simulink model "dof14model_rev"  (R2024a)
settings: Solver=ode4  StartTime=0.0  StopTime=simtime  FixedStep=samtime  RelTol=1e-3
values from neighbouring files (symbols this model uses):
  a = data(n,2)    [main_dof14model.m]
  b = data(n,3)    [main_dof14model.m]
  Csfl = data(n,22)    [main_dof14model.m]
  Csfr = data(n,23)    [main_dof14model.m]
  Csrl = data(n,24)    [main_dof14model.m]
  Csrr = data(n,25)    [main_dof14model.m]
  h = data(n,6)    [main_dof14model.m]
  Ip = data(n,10)    [main_dof14model.m]
  Ir = data(n,11)    [main_dof14model.m]
  Iw = data(n,17)    [main_dof14model.m]
  Jz = data(n,12)    [main_dof14model.m]
  Ksfl = data(n,18)    [main_dof14model.m]
  Ksfr = data(n,19)    [main_dof14model.m]
  Ksrl = data(n,20)    [main_dof14model.m]
  Ksrr = data(n,21)    [main_dof14model.m]
  Ktfl = data(n,28)    [main_dof14model.m]
  Ktfr = data(n,29)    [main_dof14model.m]
  Ktrl = data(n,30)    [main_dof14model.m]
  Ktrr = data(n,31)    [main_dof14model.m]
  Lf = data(n,8)    [main_dof14model.m]
  Lr = data(n,9)    [main_dof14model.m]
  Ms = data(n,1)    [main_dof14model.m]
  mt = data(n,7)    [main_dof14model.m]
  mufl = data(n,13)    [main_dof14model.m]
  mufr = data(n,14)    [main_dof14model.m]
  murl = data(n,15)    [main_dof14model.m]
  murr = data(n,16)    [main_dof14model.m]
  Rw = data(n,27)    [main_dof14model.m]
  wf = data(n,4)    [main_dof14model.m]
  wr = data(n,5)    [main_dof14model.m]
undefined symbols (not defined in the file or in its folder): sigbuilder_block
(part 2 of 2)

== system dof14model_rev/Subsys Tire/Subsys tfl1/Subsys Fy ==
  note: Sh
  note: x
  note: X
  note: Bx - atanBX
  note: Bx
  note: B
  alpha : Inport
  Fz : Inport  Port=2
  Bx : Product  RndMeth=Zero
  C : Constant  Value=1.3
  Divide : Product  Inputs=*/
  Product{1..4} (4 alike) : Product  RndMeth=Zero
  Scope2 : Scope
  Subsys BCD : Subsystem
  Subsys D : Subsystem
  SubsysE : Subsystem
  Subtract : Sum  Inputs=+-
  Subtract1 : Sum  Inputs=+-
  Subtract3 : Sum
  Subtract4 : Sum
  Sv : Constant  Value=0
  Sv1 : Constant  Value=0
  To Workspace1 : ToWorkspace  VariableName=Fyfrs  SampleTime=-1
  atan : Trigonometry  Operator=atan
  atanBx : Trigonometry  Operator=atan
  atanBx1 : Trigonometry
  Fy : Outport
  wires:
  Fz/1 -> SubsysE/1(Fz), Subsys D/1(Fz), Subsys BCD/1(Fz)
  alpha/1 -> Subtract4/1
  Subsys BCD/1(BCD) -> Divide/1
  Sv1/1 -> Subtract4/2
  Divide/1 -> Bx/2
  Bx/1 -> atanBx/1, Subtract1/1, Subtract/1
  atanBx/1 -> Subtract/2
  Subtract/1 -> Product1/1
  SubsysE/1(E) -> Product1/2
  Product1/1 -> Subtract1/2
  Subtract1/1 -> atan/1
  Sv/1 -> Subtract3/2
  Subtract4/1 -> Bx/1
  atan/1 -> Product3/1
  atanBx1/1 -> Product4/1
  Product3/1 -> atanBx1/1
  Product4/1 -> Subtract3/1
  Subtract3/1 -> Fy/1, To Workspace1/1, Scope2/1
  Product2/1 -> Divide/2
  Subsys D/1(D) -> Product4/2, Product2/2
  C/1 -> Product3/2, Product2/1

== system dof14model_rev/Subsys Tire/Subsys tfl1/Subsys Mz ==
  note: x
  note: X
  note: Bx - atanBX
  note: Bx
  note: B
  alpha : Inport
  Fz : Inport  Port=2
  Bx : Product  RndMeth=Zero
  C : Constant  Value=2.40
  Divide : Product  Inputs=*/
  Product{1..4} (4 alike) : Product  RndMeth=Zero
  Scope2 : Scope
  Sh2 : Constant  Value=0
  Subsys BCD : Subsystem
  Subsys D : Subsystem
  SubsysE : Subsystem
  Subtract : Sum  Inputs=+-
  Subtract1 : Sum  Inputs=+-
  Subtract3 : Sum
  Subtract4 : Sum
  Sv2 : Constant  Value=0
  To Workspace1 : ToWorkspace  VariableName=Mzfrs  SampleTime=-1
  atan : Trigonometry  Operator=atan
  atanBx : Trigonometry  Operator=atan
  atanBx1 : Trigonometry
  Mz : Outport
  wires:
  Fz/1 -> SubsysE/1(Fz), Subsys D/1(Fz), Subsys BCD/1(Fz)
  Sh2/1 -> Subtract4/2
  Divide/1 -> Bx/2
  Bx/1 -> atanBx/1, Subtract1/1, Subtract/1
  atanBx/1 -> Subtract/2
  Subtract/1 -> Product1/1
  SubsysE/1(E) -> Product1/2
  Product1/1 -> Subtract1/2
  Subtract1/1 -> atan/1
  Sv2/1 -> Subtract3/2
  Subtract4/1 -> Bx/1
  alpha/1 -> Subtract4/1
  atan/1 -> Product3/1
  atanBx1/1 -> Product4/1
  Product3/1 -> atanBx1/1
  Product4/1 -> Subtract3/1
  Subtract3/1 -> Mz/1, To Workspace1/1, Scope2/1
  Product2/1 -> Divide/2
  Subsys BCD/1(BCD) -> Divide/1
  Subsys D/1(D) -> Product4/2, Product2/2
  C/1 -> Product3/2, Product2/1

== system dof14model_rev/Subsys Tire/Subsys tfl2/Subsys Fx ==
  note: B
  note: Bx
  note: Bx - atanBX
  note: X
  note: x
  S : Inport
  Fz : Inport  Port=2
  Bx : Product  RndMeth=Zero
  C : Constant  Value=1.65
  Divide : Product  Inputs=*/
  Gain : Gain  Gain=100
  Product{1..4} (4 alike) : Product  RndMeth=Zero
  Scope2 : Scope
  Sh2 : Constant  Value=0
  Subsys BCD : Subsystem
  Subsys D : Subsystem
  SubsysE : Subsystem
  Subtract : Sum  Inputs=+-
  Subtract1 : Sum  Inputs=+-
  Subtract3 : Sum
  Subtract4 : Sum
  Sv : Constant  Value=0
  To Workspace1 : ToWorkspace  VariableName=Fxrls  SampleTime=-1
  atan : Trigonometry  Operator=atan
  atanBx : Trigonometry  Operator=atan
  atanBx1 : Trigonometry
  Fx : Outport
  wires:
  C/1 -> Product2/1, Product3/2
  Subsys D/1(D) -> Product2/2, Product4/2
  Subsys BCD/1(BCD) -> Divide/1
  Product2/1 -> Divide/2
  Subtract3/1 -> Scope2/1, To Workspace1/1, Fx/1
  Product4/1 -> Subtract3/1
  Product3/1 -> atanBx1/1
  atanBx1/1 -> Product4/1
  atan/1 -> Product3/1
  S/1 -> Gain/1
  Subtract4/1 -> Bx/1
  Sv/1 -> Subtract3/2
  Subtract1/1 -> atan/1
  Product1/1 -> Subtract1/2
  SubsysE/1(E) -> Product1/2
  Subtract/1 -> Product1/1
  atanBx/1 -> Subtract/2
  Bx/1 -> Subtract/1, Subtract1/1, atanBx/1
  Divide/1 -> Bx/2
  Sh2/1 -> Subtract4/2
  Fz/1 -> Subsys BCD/1(Fz), Subsys D/1(Fz), SubsysE/1(Fz)
  Gain/1 -> Subtract4/1

== system dof14model_rev/Subsys Tire/Subsys tfl2/Subsys Fy ==
  note: B
  note: Bx
  note: Bx - atanBX
  note: X
  note: x
  note: Sh
  alpha : Inport
  Fz : Inport  Port=2
  Bx : Product  RndMeth=Zero
  C : Constant  Value=1.3
  Divide : Product  Inputs=*/
  Product{1..4} (4 alike) : Product  RndMeth=Zero
  Scope2 : Scope
  Subsys BCD : Subsystem
  Subsys D : Subsystem
  SubsysE : Subsystem
  Subtract : Sum  Inputs=+-
  Subtract1 : Sum  Inputs=+-
  Subtract3 : Sum
  Subtract4 : Sum
  Sv : Constant  Value=0
  Sv1 : Constant  Value=0
  To Workspace1 : ToWorkspace  VariableName=Fyrls  SampleTime=-1
  atan : Trigonometry  Operator=atan
  atanBx : Trigonometry  Operator=atan
  atanBx1 : Trigonometry
  Fy : Outport
  wires:
  C/1 -> Product2/1, Product3/2
  Subsys D/1(D) -> Product2/2, Product4/2
  Product2/1 -> Divide/2
  Subtract3/1 -> Scope2/1, To Workspace1/1, Fy/1
  Product4/1 -> Subtract3/1
  Product3/1 -> atanBx1/1
  atanBx1/1 -> Product4/1
  atan/1 -> Product3/1
  Subtract4/1 -> Bx/1
  Sv/1 -> Subtract3/2
  Subtract1/1 -> atan/1
  Product1/1 -> Subtract1/2
  SubsysE/1(E) -> Product1/2
  Subtract/1 -> Product1/1
  atanBx/1 -> Subtract/2
  Bx/1 -> Subtract/1, Subtract1/1, atanBx/1
  Divide/1 -> Bx/2
  Sv1/1 -> Subtract4/2
  Subsys BCD/1(BCD) -> Divide/1
  alpha/1 -> Subtract4/1
  Fz/1 -> Subsys BCD/1(Fz), Subsys D/1(Fz), SubsysE/1(Fz)

== system dof14model_rev/Subsys Tire/Subsys tfl2/Subsys Mz ==
  note: B
  note: Bx
  note: Bx - atanBX
  note: X
  note: x
  alpha : Inport
  Fz : Inport  Port=2
  Bx : Product  RndMeth=Zero
  C : Constant  Value=2.40
  Divide : Product  Inputs=*/
  Product{1..4} (4 alike) : Product  RndMeth=Zero
  Scope2 : Scope
  Sh2 : Constant  Value=0
  Subsys BCD : Subsystem
  Subsys D : Subsystem
  SubsysE : Subsystem
  Subtract : Sum  Inputs=+-
  Subtract1 : Sum  Inputs=+-
  Subtract3 : Sum
  Subtract4 : Sum
  Sv2 : Constant  Value=0
  To Workspace1 : ToWorkspace  VariableName=Mzrls  SampleTime=-1
  atan : Trigonometry  Operator=atan
  atanBx : Trigonometry  Operator=atan
  atanBx1 : Trigonometry
  Mz : Outport
  wires:
  C/1 -> Product2/1, Product3/2
  Subsys D/1(D) -> Product2/2, Product4/2
  Subsys BCD/1(BCD) -> Divide/1
  Product2/1 -> Divide/2
  Subtract3/1 -> Scope2/1, To Workspace1/1, Mz/1
  Product4/1 -> Subtract3/1
  Product3/1 -> atanBx1/1
  atanBx1/1 -> Product4/1
  atan/1 -> Product3/1
  alpha/1 -> Subtract4/1
  Subtract4/1 -> Bx/1
  Sv2/1 -> Subtract3/2
  Subtract1/1 -> atan/1
  Product1/1 -> Subtract1/2
  SubsysE/1(E) -> Product1/2
  Subtract/1 -> Product1/1
  atanBx/1 -> Subtract/2
  Bx/1 -> Subtract/1, Subtract1/1, atanBx/1
  Divide/1 -> Bx/2
  Sh2/1 -> Subtract4/2
  Fz/1 -> Subsys BCD/1(Fz), Subsys D/1(Fz), SubsysE/1(Fz)

== system dof14model_rev/Subsys Tire/Subsys tfl3/Subsys Fx ==
  note: x
  note: X
  note: Bx - atanBX
  note: Bx
  note: B
  S : Inport
  Fz : Inport  Port=2
  Bx : Product  RndMeth=Zero
  C : Constant  Value=1.65
  Divide : Product  Inputs=*/
  Gain : Gain  Gain=100
  Product{1..4} (4 alike) : Product  RndMeth=Zero
  Scope2 : Scope
  Sh2 : Constant  Value=0
  Subsys BCD : Subsystem
  Subsys D : Subsystem
  SubsysE : Subsystem
  Subtract : Sum  Inputs=+-
  Subtract1 : Sum  Inputs=+-
  Subtract3 : Sum
  Subtract4 : Sum
  Sv : Constant  Value=0
  To Workspace1 : ToWorkspace  VariableName=Fxrrs  SampleTime=-1
  atan : Trigonometry  Operator=atan
  atanBx : Trigonometry  Operator=atan
  atanBx1 : Trigonometry
  Fx : Outport
  wires:
  Gain/1 -> Subtract4/1
  Fz/1 -> SubsysE/1(Fz), Subsys D/1(Fz), Subsys BCD/1(Fz)
  Sh2/1 -> Subtract4/2
  Divide/1 -> Bx/2
  Bx/1 -> atanBx/1, Subtract1/1, Subtract/1
  atanBx/1 -> Subtract/2
  Subtract/1 -> Product1/1
  SubsysE/1(E) -> Product1/2
  Product1/1 -> Subtract1/2
  Subtract1/1 -> atan/1
  Sv/1 -> Subtract3/2
  Subtract4/1 -> Bx/1
  S/1 -> Gain/1
  atan/1 -> Product3/1
  atanBx1/1 -> Product4/1
  Product3/1 -> atanBx1/1
  Product4/1 -> Subtract3/1
  Subtract3/1 -> Fx/1, To Workspace1/1, Scope2/1
  Product2/1 -> Divide/2
  Subsys BCD/1(BCD) -> Divide/1
  Subsys D/1(D) -> Product4/2, Product2/2
  C/1 -> Product3/2, Product2/1

== system dof14model_rev/Subsys Tire/Subsys tfl3/Subsys Fy ==
  note: Sh
  note: x
  note: X
  note: Bx - atanBX
  note: Bx
  note: B
  alpha : Inport
  Fz : Inport  Port=2
  Bx : Product  RndMeth=Zero
  C : Constant  Value=1.3
  Divide : Product  Inputs=*/
  Product{1..4} (4 alike) : Product  RndMeth=Zero
  Scope2 : Scope
  Subsys BCD : Subsystem
  Subsys D : Subsystem
  SubsysE : Subsystem
  Subtract : Sum  Inputs=+-
  Subtract1 : Sum  Inputs=+-
  Subtract3 : Sum
  Subtract4 : Sum
  Sv : Constant  Value=0
  Sv1 : Constant  Value=0
  To Workspace1 : ToWorkspace  VariableName=Fyrrs  SampleTime=-1
  atan : Trigonometry  Operator=atan
  atanBx : Trigonometry  Operator=atan
  atanBx1 : Trigonometry
  Fy : Outport
  wires:
  Fz/1 -> SubsysE/1(Fz), Subsys D/1(Fz), Subsys BCD/1(Fz)
  alpha/1 -> Subtract4/1
  Subsys BCD/1(BCD) -> Divide/1
  Sv1/1 -> Subtract4/2
  Divide/1 -> Bx/2
  Bx/1 -> atanBx/1, Subtract1/1, Subtract/1
  atanBx/1 -> Subtract/2
  Subtract/1 -> Product1/1
  SubsysE/1(E) -> Product1/2
  Product1/1 -> Subtract1/2
  Subtract1/1 -> atan/1
  Sv/1 -> Subtract3/2
  Subtract4/1 -> Bx/1
  atan/1 -> Product3/1
  atanBx1/1 -> Product4/1
  Product3/1 -> atanBx1/1
  Product4/1 -> Subtract3/1
  Subtract3/1 -> Fy/1, To Workspace1/1, Scope2/1
  Product2/1 -> Divide/2
  Subsys D/1(D) -> Product4/2, Product2/2
  C/1 -> Product3/2, Product2/1

== system dof14model_rev/Subsys Tire/Subsys tfl3/Subsys Mz ==
  note: x
  note: X
  note: Bx - atanBX
  note: Bx
  note: B
  alpha : Inport
  Fz : Inport  Port=2
  Bx : Product  RndMeth=Zero
  C : Constant  Value=2.40
  Divide : Product  Inputs=*/
  Product{1..4} (4 alike) : Product  RndMeth=Zero
  Scope2 : Scope
  Sh2 : Constant  Value=0
  Subsys BCD : Subsystem
  Subsys D : Subsystem
  SubsysE : Subsystem
  Subtract : Sum  Inputs=+-
  Subtract1 : Sum  Inputs=+-
  Subtract3 : Sum
  Subtract4 : Sum
  Sv2 : Constant  Value=0
  To Workspace1 : ToWorkspace  VariableName=Mzrrs  SampleTime=-1
  atan : Trigonometry  Operator=atan
  atanBx : Trigonometry  Operator=atan
  atanBx1 : Trigonometry
  Mz : Outport
  wires:
  Fz/1 -> SubsysE/1(Fz), Subsys D/1(Fz), Subsys BCD/1(Fz)
  Sh2/1 -> Subtract4/2
  Divide/1 -> Bx/2
  Bx/1 -> atanBx/1, Subtract1/1, Subtract/1
  atanBx/1 -> Subtract/2
  Subtract/1 -> Product1/1
  SubsysE/1(E) -> Product1/2
  Product1/1 -> Subtract1/2
  Subtract1/1 -> atan/1
  Sv2/1 -> Subtract3/2
  Subtract4/1 -> Bx/1
  alpha/1 -> Subtract4/1
  atan/1 -> Product3/1
  atanBx1/1 -> Product4/1
  Product3/1 -> atanBx1/1
  Product4/1 -> Subtract3/1
  Subtract3/1 -> Mz/1, To Workspace1/1, Scope2/1
  Product2/1 -> Divide/2
  Subsys BCD/1(BCD) -> Divide/1
  Subsys D/1(D) -> Product4/2, Product2/2
  C/1 -> Product3/2, Product2/1

== system dof14model_rev/Subsys ride/Subsys Fz/Subsys Fzfl ==
  note: mufl.g
  note: Ms.g
  note: Ms.gb
  note: a+b
  note: 2(a+b)
  note: Msg.b/2(a+b)
  Ffl : Inport
  Add : Sum
  Add1 : Sum  Inputs=+++
  Divide : Product  Inputs=*/
  Ms : Constant  Value=Ms
  Product3 : Product  RndMeth=Zero
  a : Constant  Value=a
  b : Constant  Value=b
  constant : Gain  Gain=2
  g : Gain  Gain=9.81
  g1 : Gain  Gain=9.81
  mufl : Constant  Value=mufl
  Fzfl : Outport
  wires:
  b/1 -> Product3/2, Add/1
  Product3/1 -> Divide/1
  a/1 -> Add/2
  Add/1 -> constant/1
  constant/1 -> Divide/2
  mufl/1 -> g/1
  g/1 -> Add1/2
  Ms/1 -> g1/1
  g1/1 -> Product3/1
  Divide/1 -> Add1/1
  Ffl/1 -> Add1/3
  Add1/1 -> Fzfl/1

== system dof14model_rev/Subsys ride/Subsys Fz/Subsys Fzfr ==
  note: Msg.b/2(a+b)
  note: 2(a+b)
  note: a+b
  note: Ms.gb
  note: Ms.g
  note: mufr.g
  Ffr : Inport
  Add : Sum
  Add1 : Sum  Inputs=+++
  Divide : Product  Inputs=*/
  Ms : Constant  Value=Ms
  Product3 : Product  RndMeth=Zero
  a : Constant  Value=a
  b : Constant  Value=b
  constant : Gain  Gain=2
  g : Gain  Gain=9.81
  g1 : Gain  Gain=9.81
  mufr : Constant  Value=mufr
  Fzfr : Outport
  wires:
  Add1/1 -> Fzfr/1
  Ffr/1 -> Add1/3
  Divide/1 -> Add1/1
  g1/1 -> Product3/1
  Ms/1 -> g1/1
  g/1 -> Add1/2
  mufr/1 -> g/1
  constant/1 -> Divide/2
  Add/1 -> constant/1
  a/1 -> Add/2
  Product3/1 -> Divide/1
  b/1 -> Add/1, Product3/2

== system dof14model_rev/Subsys ride/Subsys Fz/Subsys Fzrl ==
  note: Msg.a/2(a+b)
  note: 2(a+b)
  note: a+b
  note: Ms.ga
  note: Ms.g
  note: murl.g
  Frl : Inport
  Add : Sum
  Add1 : Sum  Inputs=+++
  Divide : Product  Inputs=*/
  Ms : Constant  Value=Ms
  Product3 : Product  RndMeth=Zero
  a : Constant  Value=a
  b : Constant  Value=b
  constant : Gain  Gain=2
  g : Gain  Gain=9.81
  g1 : Gain  Gain=9.81
  mufl : Constant  Value=murl
  Fzrl : Outport
  wires:
  Add1/1 -> Fzrl/1
  Frl/1 -> Add1/3
  Divide/1 -> Add1/1
  g1/1 -> Product3/1
  Ms/1 -> g1/1
  g/1 -> Add1/2
  mufl/1 -> g/1
  constant/1 -> Divide/2
  Add/1 -> constant/1
  b/1 -> Add/2
  Product3/1 -> Divide/1
  a/1 -> Add/1, Product3/2

== system dof14model_rev/Subsys ride/Subsys Fz/Subsys Fzrl1 ==
  note: murr.g
  note: Ms.g
  note: Ms.ga
  note: a+b
  note: 2(a+b)
  note: Msg.a/2(a+b)
  Frr : Inport
  Add : Sum
  Add1 : Sum  Inputs=+++
  Divide : Product  Inputs=*/
  Ms : Constant  Value=Ms
  Product3 : Product  RndMeth=Zero
  a : Constant  Value=a
  b : Constant  Value=b
  constant : Gain  Gain=2
  g : Gain  Gain=9.81
  g1 : Gain  Gain=9.81
  murr : Constant  Value=murr
  Fzrr : Outport
  wires:
  a/1 -> Product3/2, Add/1
  Product3/1 -> Divide/1
  b/1 -> Add/2
  Add/1 -> constant/1
  constant/1 -> Divide/2
  murr/1 -> g/1
  g/1 -> Add1/2
  Ms/1 -> g1/1
  g1/1 -> Product3/1
  Divide/1 -> Add1/1
  Frr/1 -> Add1/3
  Add1/1 -> Fzrr/1

== system dof14model_rev/Subsys ride/Subsys wheel fl/Ftfl ==
  Zrfl : Inport
  Zufl : Inport  Port=2
  Gain : Gain  Gain=Ktfl
  Subtract : Sum  Inputs=+-
  Ftfl : Outport
  wires:
  Subtract/1 -> Gain/1
  Zrfl/1 -> Subtract/1
  Zufl/1 -> Subtract/2
  Gain/1 -> Ftfl/1

== system dof14model_rev/Subsys ride/Subsys wheel fr/Ftfr ==
  Zrfr : Inport
  Zufr : Inport  Port=2
  Gain : Gain  Gain=Ktfr
  Subtract : Sum  Inputs=+-
  Ftfr : Outport
  wires:
  Gain/1 -> Ftfr/1
  Zufr/1 -> Subtract/2
  Zrfr/1 -> Subtract/1
  Subtract/1 -> Gain/1

== system dof14model_rev/Subsys ride/Subsys wheel rl/Ftrl ==
  Zrrl : Inport
  Zurl : Inport  Port=2
  Gain : Gain  Gain=Ktrl
  Subtract : Sum  Inputs=+-
  Ftrl : Outport
  wires:
  Subtract/1 -> Gain/1
  Zrrl/1 -> Subtract/1
  Zurl/1 -> Subtract/2
  Gain/1 -> Ftrl/1

== system dof14model_rev/Subsys ride/Subsys wheel rr/Ftfr2 ==
  Zrrr : Inport
  Zurr : Inport  Port=2
  Gain : Gain  Gain=Ktrr
  Subtract : Sum  Inputs=+-
  Ftfr : Outport
  wires:
  Gain/1 -> Ftfr/1
  Zurr/1 -> Subtract/2
  Zrrr/1 -> Subtract/1
  Subtract/1 -> Gain/1

== system dof14model_rev/Subsys Tire/Subsys tfl/Subsys Fx/Subsys BCD ==
  Fz : Inport
  Add : Sum
  Divide : Product  Inputs=*/
  Fz^1 : Math  SignedPower=on
  Fz^2 : Math  Operator=square  SignedPower=on
  Product1 : Product  RndMeth=Zero
  Product2 : Product  RndMeth=Zero
  Product3 : Product  RndMeth=Zero
  a3 : Constant  Value=49.6
  a4 : Constant  Value=226
  a5 : Constant  Value=0.069
  BCD : Outport
  wires:
  Fz/1 -> Fz^2/1, Product1/2, Product3/2
  a4/1 -> Product1/1
  a3/1 -> Product2/1
  Fz^2/1 -> Product2/2
  Product2/1 -> Add/1
  Product1/1 -> Add/2
  a5/1 -> Product3/1
  Product3/1 -> Fz^1/1
  Add/1 -> Divide/1
  Fz^1/1 -> Divide/2
  Divide/1 -> BCD/1

== system dof14model_rev/Subsys Tire/Subsys tfl/Subsys Fx/Subsys D ==
  Fz : Inport
  Add1 : Sum
  Fz^2 : Math  Operator=square  SignedPower=on
  Product : Product  RndMeth=Zero
  Product1 : Product  RndMeth=Zero
  a1 : Constant  Value=-21.3
  a2 : Constant  Value=1144
  D : Outport
  wires:
  Fz/1 -> Fz^2/1, Product1/2
  a1/1 -> Product/1
  Fz^2/1 -> Product/2
  a2/1 -> Product1/1
  Product1/1 -> Add1/2
  Product/1 -> Add1/1
  Add1/1 -> D/1

== system dof14model_rev/Subsys Tire/Subsys tfl/Subsys Fx/SubsysE ==
  Fz : Inport
  Add : Sum  Inputs=+++
  Fz^2 : Math  Operator=square  SignedPower=on
  Product1 : Product  RndMeth=Zero
  Product3 : Product  RndMeth=Zero
  a6 : Constant  Value=-0.006
  a7 : Constant  Value=0.056
  a8 : Constant  Value=0.486
  E : Outport
  wires:
  Fz/1 -> Fz^2/1, Product1/2
  a7/1 -> Product1/1
  a6/1 -> Product3/1
  Fz^2/1 -> Product3/2
  Product3/1 -> Add/1
  Product1/1 -> Add/2
  Add/1 -> E/1
  a8/1 -> Add/3

== system dof14model_rev/Subsys Tire/Subsys tfl/Subsys Fy/Subsys BCD ==
  Fz : Inport
  Product1 : Product  RndMeth=Zero
  Product2 : Product  RndMeth=Zero
  Product3 : Product  RndMeth=Zero
  Trigonometric Function : Trigonometry  Operator=atan
  Trigonometric Function1 : Trigonometry
  a3 : Constant  Value=1078
  a4 : Constant  Value=1.82
  a5 : Constant  Value=0.208
  BCD : Outport
  wires:
  Fz/1 -> Product2/2
  a5/1 -> Product2/1
  Product2/1 -> Trigonometric Function/1
  Trigonometric Function/1 -> Product1/2
  a4/1 -> Product1/1
  Product1/1 -> Trigonometric Function1/1
  Trigonometric Function1/1 -> Product3/2
  a3/1 -> Product3/1
  Product3/1 -> BCD/1

== system dof14model_rev/Subsys Tire/Subsys tfl/Subsys Fy/Subsys D ==
  Fz : Inport
  Add1 : Sum
  Fz^2 : Math  Operator=square  SignedPower=on
  Product : Product  RndMeth=Zero
  Product1 : Product  RndMeth=Zero
  a1 : Constant  Value=-22.1
  a2 : Constant  Value=1011
  D : Outport
  wires:
  Fz/1 -> Fz^2/1, Product1/2
  a1/1 -> Product/1
  Fz^2/1 -> Product/2
  a2/1 -> Product1/1
  Product1/1 -> Add1/2
  Product/1 -> Add1/1
  Add1/1 -> D/1

== system dof14model_rev/Subsys Tire/Subsys tfl/Subsys Fy/SubsysE ==
  Fz : Inport
  Add : Sum  Inputs=+++
  Fz^2 : Math  Operator=square  SignedPower=on
  Product1 : Product  RndMeth=Zero
  Product3 : Product  RndMeth=Zero
  a6 : Constant  Value=0.0000
  a7 : Constant  Value=-0.354
  a8 : Constant  Value=0.707
  E : Outport
  wires:
  Fz/1 -> Fz^2/1, Product1/2
  a7/1 -> Product1/1
  a6/1 -> Product3/1
  Fz^2/1 -> Product3/2
  Product3/1 -> Add/1
  Product1/1 -> Add/2
  Add/1 -> E/1
  a8/1 -> Add/3

== system dof14model_rev/Subsys Tire/Subsys tfl/Subsys Mz/Subsys BCD ==
  Fz : Inport
  Add : Sum
  Divide : Product  Inputs=*/
  Fz^1 : Math  SignedPower=on
  Fz^2 : Math  Operator=square  SignedPower=on
  Product1 : Product  RndMeth=Zero
  Product2 : Product  RndMeth=Zero
  Product3 : Product  RndMeth=Zero
  a3 : Constant  Value=-1.86
  a4 : Constant  Value=-2.73
  a5 : Constant  Value=0.110
  BCD : Outport
  wires:
  Fz/1 -> Fz^2/1, Product1/2, Product3/2
  a4/1 -> Product1/1
  a3/1 -> Product2/1
  Fz^2/1 -> Product2/2
  Product2/1 -> Add/1
  Product1/1 -> Add/2
  a5/1 -> Product3/1
  Product3/1 -> Fz^1/1
  Add/1 -> Divide/1
  Fz^1/1 -> Divide/2
  Divide/1 -> BCD/1

== system dof14model_rev/Subsys Tire/Subsys tfl/Subsys Mz/Subsys D ==
  Fz : Inport
  Add1 : Sum
  Fz^2 : Math  Operator=square  SignedPower=on
  Product : Product  RndMeth=Zero
  Product1 : Product  RndMeth=Zero
  a1 : Constant  Value=-2.72
  a2 : Constant  Value=-2.28
  D : Outport
  wires:
  Fz/1 -> Fz^2/1, Product1/2
  a1/1 -> Product/1
  Fz^2/1 -> Product/2
  a2/1 -> Product1/1
  Product1/1 -> Add1/2
  Product/1 -> Add1/1
  Add1/1 -> D/1

== system dof14model_rev/Subsys Tire/Subsys tfl/Subsys Mz/SubsysE ==
  Fz : Inport
  Add : Sum  Inputs=+++
  Fz^2 : Math  Operator=square  SignedPower=on
  Product1 : Product  RndMeth=Zero
  Product3 : Product  RndMeth=Zero
  a6 : Constant  Value=-0.070
  a7 : Constant  Value=0.643
  a8 : Constant  Value=-4.04
  E : Outport
  wires:
  Fz/1 -> Fz^2/1, Product1/2
  a7/1 -> Product1/1
  a6/1 -> Product3/1
  Fz^2/1 -> Product3/2
  Product3/1 -> Add/1
  Product1/1 -> Add/2
  Add/1 -> E/1
  a8/1 -> Add/3

== system dof14model_rev/Subsys Tire/Subsys tfl1/Subsys Fx/Subsys BCD ==
  Fz : Inport
  Add : Sum
  Divide : Product  Inputs=*/
  Fz^1 : Math  SignedPower=on
  Fz^2 : Math  Operator=square  SignedPower=on
  Product1 : Product  RndMeth=Zero
  Product2 : Product  RndMeth=Zero
  Product3 : Product  RndMeth=Zero
  a3 : Constant  Value=49.6
  a4 : Constant  Value=226
  a5 : Constant  Value=0.069
  BCD : Outport
  wires:
  Divide/1 -> BCD/1
  Fz^1/1 -> Divide/2
  Add/1 -> Divide/1
  Product3/1 -> Fz^1/1
  a5/1 -> Product3/1
  Product1/1 -> Add/2
  Product2/1 -> Add/1
  Fz^2/1 -> Product2/2
  a3/1 -> Product2/1
  a4/1 -> Product1/1
  Fz/1 -> Product3/2, Product1/2, Fz^2/1

== system dof14model_rev/Subsys Tire/Subsys tfl1/Subsys Fx/Subsys D ==
  Fz : Inport
  Add1 : Sum
  Fz^2 : Math  Operator=square  SignedPower=on
  Product : Product  RndMeth=Zero
  Product1 : Product  RndMeth=Zero
  a1 : Constant  Value=-21.3
  a2 : Constant  Value=1144
  D : Outport
  wires:
  Add1/1 -> D/1
  Product/1 -> Add1/1
  Product1/1 -> Add1/2
  a2/1 -> Product1/1
  Fz^2/1 -> Product/2
  a1/1 -> Product/1
  Fz/1 -> Product1/2, Fz^2/1

== system dof14model_rev/Subsys Tire/Subsys tfl1/Subsys Fx/SubsysE ==
  Fz : Inport
  Add : Sum  Inputs=+++
  Fz^2 : Math  Operator=square  SignedPower=on
  Product1 : Product  RndMeth=Zero
  Product3 : Product  RndMeth=Zero
  a6 : Constant  Value=-0.006
  a7 : Constant  Value=0.056
  a8 : Constant  Value=0.486
  E : Outport
  wires:
  a8/1 -> Add/3
  Add/1 -> E/1
  Product1/1 -> Add/2
  Product3/1 -> Add/1
  Fz^2/1 -> Product3/2
  a6/1 -> Product3/1
  a7/1 -> Product1/1
  Fz/1 -> Product1/2, Fz^2/1

== system dof14model_rev/Subsys Tire/Subsys tfl1/Subsys Fy/Subsys BCD ==
  Fz : Inport
  Product1 : Product  RndMeth=Zero
  Product2 : Product  RndMeth=Zero
  Product3 : Product  RndMeth=Zero
  Trigonometric Function : Trigonometry  Operator=atan
  Trigonometric Function1 : Trigonometry
  a3 : Constant  Value=1078
  a4 : Constant  Value=1.82
  a5 : Constant  Value=0.208
  BCD : Outport
  wires:
  Product3/1 -> BCD/1
  a3/1 -> Product3/1
  Trigonometric Function1/1 -> Product3/2
  Product1/1 -> Trigonometric Function1/1
  a4/1 -> Product1/1
  Trigonometric Function/1 -> Product1/2
  Product2/1 -> Trigonometric Function/1
  a5/1 -> Product2/1
  Fz/1 -> Product2/2

== system dof14model_rev/Subsys Tire/Subsys tfl1/Subsys Fy/Subsys D ==
  Fz : Inport
  Add1 : Sum
  Fz^2 : Math  Operator=square  SignedPower=on
  Product : Product  RndMeth=Zero
  Product1 : Product  RndMeth=Zero
  a1 : Constant  Value=-22.1
  a2 : Constant  Value=1011
  D : Outport
  wires:
  Add1/1 -> D/1
  Product/1 -> Add1/1
  Product1/1 -> Add1/2
  a2/1 -> Product1/1
  Fz^2/1 -> Product/2
  a1/1 -> Product/1
  Fz/1 -> Product1/2, Fz^2/1

== system dof14model_rev/Subsys Tire/Subsys tfl1/Subsys Fy/SubsysE ==
  Fz : Inport
  Add : Sum  Inputs=+++
  Fz^2 : Math  Operator=square  SignedPower=on
  Product1 : Product  RndMeth=Zero
  Product3 : Product  RndMeth=Zero
  a6 : Constant  Value=0.0000
  a7 : Constant  Value=-0.354
  a8 : Constant  Value=0.707
  E : Outport
  wires:
  a8/1 -> Add/3
  Add/1 -> E/1
  Product1/1 -> Add/2
  Product3/1 -> Add/1
  Fz^2/1 -> Product3/2
  a6/1 -> Product3/1
  a7/1 -> Product1/1
  Fz/1 -> Product1/2, Fz^2/1

== system dof14model_rev/Subsys Tire/Subsys tfl1/Subsys Mz/Subsys BCD ==
  Fz : Inport
  Add : Sum
  Divide : Product  Inputs=*/
  Fz^1 : Math  SignedPower=on
  Fz^2 : Math  Operator=square  SignedPower=on
  Product1 : Product  RndMeth=Zero
  Product2 : Product  RndMeth=Zero
  Product3 : Product  RndMeth=Zero
  a3 : Constant  Value=-1.86
  a4 : Constant  Value=-2.73
  a5 : Constant  Value=0.110
  BCD : Outport
  wires:
  Divide/1 -> BCD/1
  Fz^1/1 -> Divide/2
  Add/1 -> Divide/1
  Product3/1 -> Fz^1/1
  a5/1 -> Product3/1
  Product1/1 -> Add/2
  Product2/1 -> Add/1
  Fz^2/1 -> Product2/2
  a3/1 -> Product2/1
  a4/1 -> Product1/1
  Fz/1 -> Product3/2, Product1/2, Fz^2/1

== system dof14model_rev/Subsys Tire/Subsys tfl1/Subsys Mz/Subsys D ==
  Fz : Inport
  Add1 : Sum
  Fz^2 : Math  Operator=square  SignedPower=on
  Product : Product  RndMeth=Zero
  Product1 : Product  RndMeth=Zero
  a1 : Constant  Value=-2.72
  a2 : Constant  Value=-2.28
  D : Outport
  wires:
  Add1/1 -> D/1
  Product/1 -> Add1/1
  Product1/1 -> Add1/2
  a2/1 -> Product1/1
  Fz^2/1 -> Product/2
  a1/1 -> Product/1
  Fz/1 -> Product1/2, Fz^2/1

== system dof14model_rev/Subsys Tire/Subsys tfl1/Subsys Mz/SubsysE ==
  Fz : Inport
  Add : Sum  Inputs=+++
  Fz^2 : Math  Operator=square  SignedPower=on
  Product1 : Product  RndMeth=Zero
  Product3 : Product  RndMeth=Zero
  a6 : Constant  Value=-0.070
  a7 : Constant  Value=0.643
  a8 : Constant  Value=-4.04
  E : Outport
  wires:
  a8/1 -> Add/3
  Add/1 -> E/1
  Product1/1 -> Add/2
  Product3/1 -> Add/1
  Fz^2/1 -> Product3/2
  a6/1 -> Product3/1
  a7/1 -> Product1/1
  Fz/1 -> Product1/2, Fz^2/1

== system dof14model_rev/Subsys Tire/Subsys tfl2/Subsys Fx/Subsys BCD ==
  Fz : Inport
  Add : Sum
  Divide : Product  Inputs=*/
  Fz^1 : Math  SignedPower=on
  Fz^2 : Math  Operator=square  SignedPower=on
  Product1 : Product  RndMeth=Zero
  Product2 : Product  RndMeth=Zero
  Product3 : Product  RndMeth=Zero
  a3 : Constant  Value=49.6
  a4 : Constant  Value=226
  a5 : Constant  Value=0.069
  BCD : Outport
  wires:
  Fz/1 -> Fz^2/1, Product1/2, Product3/2
  a4/1 -> Product1/1
  a3/1 -> Product2/1
  Fz^2/1 -> Product2/2
  Product2/1 -> Add/1
  Product1/1 -> Add/2
  a5/1 -> Product3/1
  Product3/1 -> Fz^1/1
  Add/1 -> Divide/1
  Fz^1/1 -> Divide/2
  Divide/1 -> BCD/1

== system dof14model_rev/Subsys Tire/Subsys tfl2/Subsys Fx/Subsys D ==
  Fz : Inport
  Add1 : Sum
  Fz^2 : Math  Operator=square  SignedPower=on
  Product : Product  RndMeth=Zero
  Product1 : Product  RndMeth=Zero
  a1 : Constant  Value=-21.3
  a2 : Constant  Value=1144
  D : Outport
  wires:
  Fz/1 -> Fz^2/1, Product1/2
  a1/1 -> Product/1
  Fz^2/1 -> Product/2
  a2/1 -> Product1/1
  Product1/1 -> Add1/2
  Product/1 -> Add1/1
  Add1/1 -> D/1

== system dof14model_rev/Subsys Tire/Subsys tfl2/Subsys Fx/SubsysE ==
  Fz : Inport
  Add : Sum  Inputs=+++
  Fz^2 : Math  Operator=square  SignedPower=on
  Product1 : Product  RndMeth=Zero
  Product3 : Product  RndMeth=Zero
  a6 : Constant  Value=-0.006
  a7 : Constant  Value=0.056
  a8 : Constant  Value=0.486
  E : Outport
  wires:
  Fz/1 -> Fz^2/1, Product1/2
  a7/1 -> Product1/1
  a6/1 -> Product3/1
  Fz^2/1 -> Product3/2
  Product3/1 -> Add/1
  Product1/1 -> Add/2
  Add/1 -> E/1
  a8/1 -> Add/3

== system dof14model_rev/Subsys Tire/Subsys tfl2/Subsys Fy/Subsys BCD ==
  Fz : Inport
  Product1 : Product  RndMeth=Zero
  Product2 : Product  RndMeth=Zero
  Product3 : Product  RndMeth=Zero
  Trigonometric Function : Trigonometry  Operator=atan
  Trigonometric Function1 : Trigonometry
  a3 : Constant  Value=1078
  a4 : Constant  Value=1.82
  a5 : Constant  Value=0.208
  BCD : Outport
  wires:
  Fz/1 -> Product2/2
  a5/1 -> Product2/1
  Product2/1 -> Trigonometric Function/1
  Trigonometric Function/1 -> Product1/2
  a4/1 -> Product1/1
  Product1/1 -> Trigonometric Function1/1
  Trigonometric Function1/1 -> Product3/2
  a3/1 -> Product3/1
  Product3/1 -> BCD/1

== system dof14model_rev/Subsys Tire/Subsys tfl2/Subsys Fy/Subsys D ==
  Fz : Inport
  Add1 : Sum
  Fz^2 : Math  Operator=square  SignedPower=on
  Product : Product  RndMeth=Zero
  Product1 : Product  RndMeth=Zero
  a1 : Constant  Value=-22.1
  a2 : Constant  Value=1011
  D : Outport
  wires:
  Fz/1 -> Fz^2/1, Product1/2
  a1/1 -> Product/1
  Fz^2/1 -> Product/2
  a2/1 -> Product1/1
  Product1/1 -> Add1/2
  Product/1 -> Add1/1
  Add1/1 -> D/1

== system dof14model_rev/Subsys Tire/Subsys tfl2/Subsys Fy/SubsysE ==
  Fz : Inport
  Add : Sum  Inputs=+++
  Fz^2 : Math  Operator=square  SignedPower=on
  Product1 : Product  RndMeth=Zero
  Product3 : Product  RndMeth=Zero
  a6 : Constant  Value=0.0000
  a7 : Constant  Value=-0.354
  a8 : Constant  Value=0.707
  E : Outport
  wires:
  Fz/1 -> Fz^2/1, Product1/2
  a7/1 -> Product1/1
  a6/1 -> Product3/1
  Fz^2/1 -> Product3/2
  Product3/1 -> Add/1
  Product1/1 -> Add/2
  Add/1 -> E/1
  a8/1 -> Add/3

== system dof14model_rev/Subsys Tire/Subsys tfl2/Subsys Mz/Subsys BCD ==
  Fz : Inport
  Add : Sum
  Divide : Product  Inputs=*/
  Fz^1 : Math  SignedPower=on
  Fz^2 : Math  Operator=square  SignedPower=on
  Product1 : Product  RndMeth=Zero
  Product2 : Product  RndMeth=Zero
  Product3 : Product  RndMeth=Zero
  a3 : Constant  Value=-1.86
  a4 : Constant  Value=-2.73
  a5 : Constant  Value=0.110
  BCD : Outport
  wires:
  Fz/1 -> Fz^2/1, Product1/2, Product3/2
  a4/1 -> Product1/1
  a3/1 -> Product2/1
  Fz^2/1 -> Product2/2
  Product2/1 -> Add/1
  Product1/1 -> Add/2
  a5/1 -> Product3/1
  Product3/1 -> Fz^1/1
  Add/1 -> Divide/1
  Fz^1/1 -> Divide/2
  Divide/1 -> BCD/1

== system dof14model_rev/Subsys Tire/Subsys tfl2/Subsys Mz/Subsys D ==
  Fz : Inport
  Add1 : Sum
  Fz^2 : Math  Operator=square  SignedPower=on
  Product : Product  RndMeth=Zero
  Product1 : Product  RndMeth=Zero
  a1 : Constant  Value=-2.72
  a2 : Constant  Value=-2.28
  D : Outport
  wires:
  Fz/1 -> Fz^2/1, Product1/2
  a1/1 -> Product/1
  Fz^2/1 -> Product/2
  a2/1 -> Product1/1
  Product1/1 -> Add1/2
  Product/1 -> Add1/1
  Add1/1 -> D/1

== system dof14model_rev/Subsys Tire/Subsys tfl2/Subsys Mz/SubsysE ==
  Fz : Inport
  Add : Sum  Inputs=+++
  Fz^2 : Math  Operator=square  SignedPower=on
  Product1 : Product  RndMeth=Zero
  Product3 : Product  RndMeth=Zero
  a6 : Constant  Value=-0.070
  a7 : Constant  Value=0.643
  a8 : Constant  Value=-4.04
  E : Outport
  wires:
  Fz/1 -> Fz^2/1, Product1/2
  a7/1 -> Product1/1
  a6/1 -> Product3/1
  Fz^2/1 -> Product3/2
  Product3/1 -> Add/1
  Product1/1 -> Add/2
  Add/1 -> E/1
  a8/1 -> Add/3

== system dof14model_rev/Subsys Tire/Subsys tfl3/Subsys Fx/Subsys BCD ==
  Fz : Inport
  Add : Sum
  Divide : Product  Inputs=*/
  Fz^1 : Math  SignedPower=on
  Fz^2 : Math  Operator=square  SignedPower=on
  Product1 : Product  RndMeth=Zero
  Product2 : Product  RndMeth=Zero
  Product3 : Product  RndMeth=Zero
  a3 : Constant  Value=49.6
  a4 : Constant  Value=226
  a5 : Constant  Value=0.069
  BCD : Outport
  wires:
  Divide/1 -> BCD/1
  Fz^1/1 -> Divide/2
  Add/1 -> Divide/1
  Product3/1 -> Fz^1/1
  a5/1 -> Product3/1
  Product1/1 -> Add/2
  Product2/1 -> Add/1
  Fz^2/1 -> Product2/2
  a3/1 -> Product2/1
  a4/1 -> Product1/1
  Fz/1 -> Product3/2, Product1/2, Fz^2/1

== system dof14model_rev/Subsys Tire/Subsys tfl3/Subsys Fx/Subsys D ==
  Fz : Inport
  Add1 : Sum
  Fz^2 : Math  Operator=square  SignedPower=on
  Product : Product  RndMeth=Zero
  Product1 : Product  RndMeth=Zero
  a1 : Constant  Value=-21.3
  a2 : Constant  Value=1144
  D : Outport
  wires:
  Add1/1 -> D/1
  Product/1 -> Add1/1
  Product1/1 -> Add1/2
  a2/1 -> Product1/1
  Fz^2/1 -> Product/2
  a1/1 -> Product/1
  Fz/1 -> Product1/2, Fz^2/1

== system dof14model_rev/Subsys Tire/Subsys tfl3/Subsys Fx/SubsysE ==
  Fz : Inport
  Add : Sum  Inputs=+++
  Fz^2 : Math  Operator=square  SignedPower=on
  Product1 : Product  RndMeth=Zero
  Product3 : Product  RndMeth=Zero
  a6 : Constant  Value=-0.006
  a7 : Constant  Value=0.056
  a8 : Constant  Value=0.486
  E : Outport
  wires:
  a8/1 -> Add/3
  Add/1 -> E/1
  Product1/1 -> Add/2
  Product3/1 -> Add/1
  Fz^2/1 -> Product3/2
  a6/1 -> Product3/1
  a7/1 -> Product1/1
  Fz/1 -> Product1/2, Fz^2/1

== system dof14model_rev/Subsys Tire/Subsys tfl3/Subsys Fy/Subsys BCD ==
  Fz : Inport
  Product1 : Product  RndMeth=Zero
  Product2 : Product  RndMeth=Zero
  Product3 : Product  RndMeth=Zero
  Trigonometric Function : Trigonometry  Operator=atan
  Trigonometric Function1 : Trigonometry
  a3 : Constant  Value=1078
  a4 : Constant  Value=1.82
  a5 : Constant  Value=0.208
  BCD : Outport
  wires:
  Product3/1 -> BCD/1
  a3/1 -> Product3/1
  Trigonometric Function1/1 -> Product3/2
  Product1/1 -> Trigonometric Function1/1
  a4/1 -> Product1/1
  Trigonometric Function/1 -> Product1/2
  Product2/1 -> Trigonometric Function/1
  a5/1 -> Product2/1
  Fz/1 -> Product2/2

== system dof14model_rev/Subsys Tire/Subsys tfl3/Subsys Fy/Subsys D ==
  Fz : Inport
  Add1 : Sum
  Fz^2 : Math  Operator=square  SignedPower=on
  Product : Product  RndMeth=Zero
  Product1 : Product  RndMeth=Zero
  a1 : Constant  Value=-22.1
  a2 : Constant  Value=1011
  D : Outport
  wires:
  Add1/1 -> D/1
  Product/1 -> Add1/1
  Product1/1 -> Add1/2
  a2/1 -> Product1/1
  Fz^2/1 -> Product/2
  a1/1 -> Product/1
  Fz/1 -> Product1/2, Fz^2/1

== system dof14model_rev/Subsys Tire/Subsys tfl3/Subsys Fy/SubsysE ==
  Fz : Inport
  Add : Sum  Inputs=+++
  Fz^2 : Math  Operator=square  SignedPower=on
  Product1 : Product  RndMeth=Zero
  Product3 : Product  RndMeth=Zero
  a6 : Constant  Value=0.0000
  a7 : Constant  Value=-0.354
  a8 : Constant  Value=0.707
  E : Outport
  wires:
  a8/1 -> Add/3
  Add/1 -> E/1
  Product1/1 -> Add/2
  Product3/1 -> Add/1
  Fz^2/1 -> Product3/2
  a6/1 -> Product3/1
  a7/1 -> Product1/1
  Fz/1 -> Product1/2, Fz^2/1

== system dof14model_rev/Subsys Tire/Subsys tfl3/Subsys Mz/Subsys BCD ==
  Fz : Inport
  Add : Sum
  Divide : Product  Inputs=*/
  Fz^1 : Math  SignedPower=on
  Fz^2 : Math  Operator=square  SignedPower=on
  Product1 : Product  RndMeth=Zero
  Product2 : Product  RndMeth=Zero
  Product3 : Product  RndMeth=Zero
  a3 : Constant  Value=-1.86
  a4 : Constant  Value=-2.73
  a5 : Constant  Value=0.110
  BCD : Outport
  wires:
  Divide/1 -> BCD/1
  Fz^1/1 -> Divide/2
  Add/1 -> Divide/1
  Product3/1 -> Fz^1/1
  a5/1 -> Product3/1
  Product1/1 -> Add/2
  Product2/1 -> Add/1
  Fz^2/1 -> Product2/2
  a3/1 -> Product2/1
  a4/1 -> Product1/1
  Fz/1 -> Product3/2, Product1/2, Fz^2/1

== system dof14model_rev/Subsys Tire/Subsys tfl3/Subsys Mz/Subsys D ==
  Fz : Inport
  Add1 : Sum
  Fz^2 : Math  Operator=square  SignedPower=on
  Product : Product  RndMeth=Zero
  Product1 : Product  RndMeth=Zero
  a1 : Constant  Value=-2.72
  a2 : Constant  Value=-2.28
  D : Outport
  wires:
  Add1/1 -> D/1
  Product/1 -> Add1/1
  Product1/1 -> Add1/2
  a2/1 -> Product1/1
  Fz^2/1 -> Product/2
  a1/1 -> Product/1
  Fz/1 -> Product1/2, Fz^2/1

== system dof14model_rev/Subsys Tire/Subsys tfl3/Subsys Mz/SubsysE ==
  Fz : Inport
  Add : Sum  Inputs=+++
  Fz^2 : Math  Operator=square  SignedPower=on
  Product1 : Product  RndMeth=Zero
  Product3 : Product  RndMeth=Zero
  a6 : Constant  Value=-0.070
  a7 : Constant  Value=0.643
  a8 : Constant  Value=-4.04
  E : Outport
  wires:
  a8/1 -> Add/3
  Add/1 -> E/1
  Product1/1 -> Add/2
  Product3/1 -> Add/1
  Fz^2/1 -> Product3/2
  a6/1 -> Product3/1
  a7/1 -> Product1/1
  Fz/1 -> Product1/2, Fz^2/1

== matlab function dof14model_rev/Subsys Handling/MATLAB Function ==
  data: vx input; beta output; vy input
function beta = fcn(vx,vy)

beta = atan2(vy,vx);
